simulink model "mashfazy"  (Simulink 7.6)
settings: Solver=ode45  StartTime=0.0  StopTime=60.0  RelTol=1e-3
libraries: simulink x1
settings Model: Creator=jahangir_ins  LastModifiedBy=saleh
settings DebuggingCC: StrictBusMsg=Warning

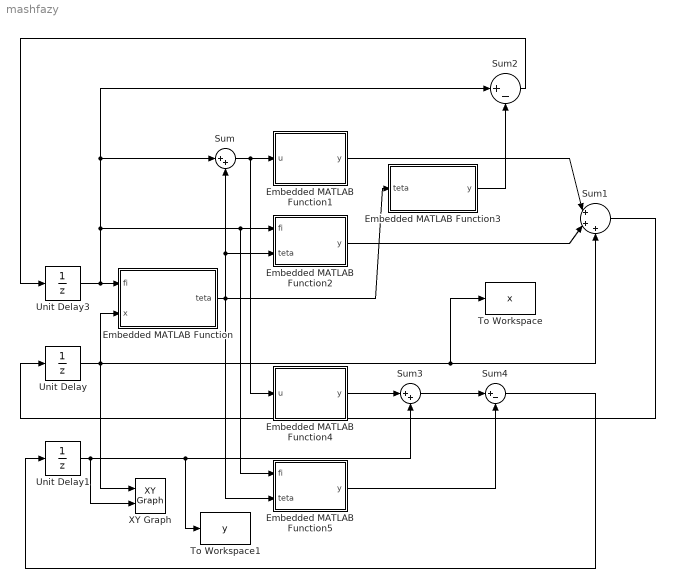
== system mashfazy ==
  Embedded MATLAB Function : Stateflow chart  TreatAsAtomicUnit=on
  Embedded MATLAB Function1 : Stateflow chart  TreatAsAtomicUnit=on
  Embedded MATLAB Function2 : Stateflow chart  TreatAsAtomicUnit=on
  Embedded MATLAB Function3 : Stateflow chart  TreatAsAtomicUnit=on
  Embedded MATLAB Function4 : Stateflow chart  TreatAsAtomicUnit=on
  Embedded MATLAB Function5 : Stateflow chart  TreatAsAtomicUnit=on
  Sum : Sum  Inputs=|++  SampleTime=.1
  Sum1 : Sum  Inputs=|+++  SampleTime=.1
  Sum2 : Sum  Inputs=|+-  SampleTime=.1
  Sum3 : Sum  Inputs=|++  SampleTime=.1
  Sum4 : Sum  Inputs=|+-  SampleTime=.1
  To Workspace : ToWorkspace  VariableName=x  SampleTime=.1  SaveFormat=Array
  To Workspace1 : ToWorkspace  VariableName=y  SampleTime=.1  SaveFormat=Array
  Unit Delay : UnitDelay  X0=17  SampleTime=.1
  Unit Delay1 : UnitDelay  X0=1  SampleTime=.1
  Unit Delay3 : UnitDelay  X0=-40  SampleTime=.1
  XY Graph : simulink/Sinks/XY Graph  SystemSampleTime=-1  xmin=0  xmax=25  ymin=-10  ymax=50  st=.1
  wires:
  Embedded MATLAB Function/1(teta) -> Embedded MATLAB Function3/1(teta), Embedded MATLAB Function2/2(teta), Sum/2, Embedded MATLAB Function5/2(teta)
  Unit Delay3/1 -> Embedded MATLAB Function/1(fi), Sum2/1, Sum/1, Embedded MATLAB Function2/1(fi), Embedded MATLAB Function5/1(fi)
  Sum/1 -> Embedded MATLAB Function1/1(u), Embedded MATLAB Function4/1(u)
  Embedded MATLAB Function1/1(y) -> Sum1/1
  Unit Delay/1 -> Embedded MATLAB Function/2(x), Sum1/3, To Workspace/1, XY Graph/1
  Embedded MATLAB Function2/1(y) -> Sum1/2
  Embedded MATLAB Function3/1(y) -> Sum2/2
  Sum2/1 -> Unit Delay3/1
  Sum1/1 -> Unit Delay/1
  Embedded MATLAB Function4/1(y) -> Sum3/1
  Unit Delay1/1 -> XY Graph/2, Sum3/2, To Workspace1/1
  Sum3/1 -> Sum4/1
  Embedded MATLAB Function5/1(y) -> Sum4/2
  Sum4/1 -> Unit Delay1/1

== matlab function Embedded MATLAB Function1 ==
  data: u input double; y output double
function y = func1(u)
u=u*(pi/180);
y=cos(u);

== matlab function Embedded MATLAB Function ==
  data: fi input double; teta output double; x input double
function teta=mashin2(fi,x)
sum1=0;sum2=0;
y=[-26.6   -40    0     0     0;
   -26.6    -40   -40   -40   -40;
    13.3 -13.3  -26.6   -40 -26.6;
    26.6  26.6     0  -26.6 -26.6;
    26.6     40  26.6  13.3 -13.3;
    0        40    40    40  26.6;
    0        0     0     40  26.6];
t=[ 1  1  0  0  0;
    1  1  1  1  1;
    1  1  1  1  1;
    1  1  1  1  1;
    1  1  1  1  1;
    0  1  1  1  1;
    0  0  0  1  1];
a=-45;
for i=1:7
    if abs(fi-a)<=45
       r=1-(abs(fi-a)/45);
    else
       r=0;
    end
    a=a+45;
    b=2;
    for j=1:5
        if abs(x-b)<=4
           s=1-(abs(x-b)/4);
        else
           s=0;
        end
    b=b+4;
    c1=r*s*y(i,j);
    sum1=sum1+c1;
    c2=r*s*t(i,j);
    sum2=sum2+c2;
    end
end
teta=sum1/sum2;
end

== matlab function Embedded MATLAB Function2 ==
  data: fi input double; y output double; teta input double
function y = func2(fi,teta)
fi=fi*(pi/180);
teta=teta*(pi/180);
y=sin(fi)*sin(teta);

== matlab function Embedded MATLAB Function3 ==
  data: teta input double; y output double
function y = fanc5(teta)
teta=teta*(pi/180);
teta=asin(.5*sin(teta));
y=(180/pi)*teta;

== matlab function Embedded MATLAB Function4 ==
  data: u input double; y output double
function y = func3(u)
u=u*(pi/180);
y=sin(u);

== matlab function Embedded MATLAB Function5 ==
  data: fi input double; y output double; teta input double
function y = func4(fi,teta)
fi=fi*(pi/180);
teta=teta*(pi/180);
y=cos(fi)*sin(teta);
